simulink model "F18_Trim_2016b"  (R2016b)
settings: Solver=ode45  StartTime=0.0  StopTime=10.0  RelTol=1e-3  EnableMultiTasking=on
settings Model: Creator=mpc5200  LastModifiedBy=User
settings DataIOCC: LimitDataPoints=on  SaveFormat=Array  SignalLoggingSaveFormat=ModelDataLogs
settings OptimizationCC: ExpressionDepthLimit=2147483647  InitFltsAndDblsToZero=on  LifeSpan=inf
settings DebuggingCC: AlgebraicLoopMsg=none  SaveWithParameterizedLinksMsg=none  UnderspecifiedInitializationDetection=Classic  MergeDetectMultiDrivingBlocksExec=none  FcnCallInpInsideContextMsg=warning  UnconnectedInputMsg=none  UnconnectedOutputMsg=none  UnconnectedLineMsg=none  StateNameClashWarn=warning  SFUnexpectedBacktrackingDiag=warning  SFNoUnconditionalDefaultTransitionDiag=warning  SFExecutionAtInitializationDiag=none
settings HardwareCC: ProdBitPerPointer=32  ProdBitPerSizeT=32  ProdBitPerPtrDiffT=32  ProdLargestAtomicFloat=None  ProdIntDivRoundTo=Undefined  ProdEndianess=Unspecified  ProdWordSize=32  ProdHWDeviceType=32-bit Generic
settings ModelReferenceCC: PropagateSignalLabelsOutOfModel=off
settings GRTTargetCC: TargetFcnLib=ansi_tfl_tmw.mat  TargetLangStandard=C89/C90 (ANSI)  CombineOutputUpdateFcns=off  GRTInterface=on
settings ConfigComp: CovMetricSettings=dw  CovHtmlReporting=on  CovSaveCumulativeToWorkspaceVar=on  CovSaveSingleToWorkspaceVar=on  CovExternalEMLEnable=off

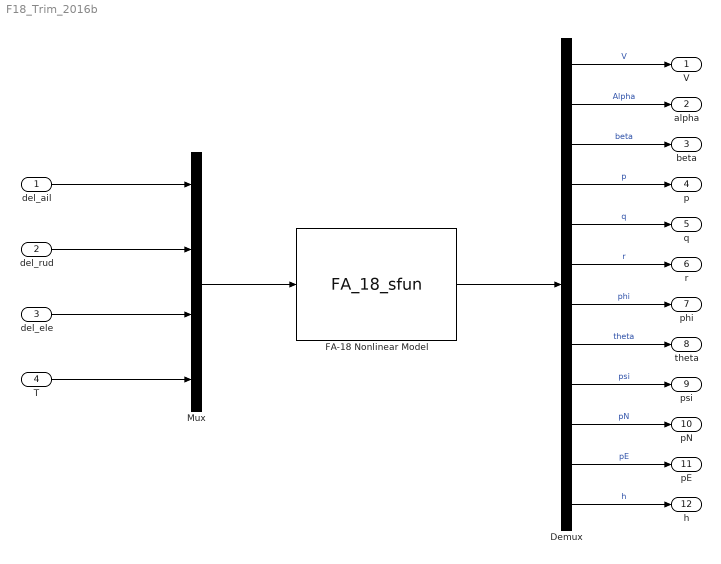
== system F18_Trim_2016b ==
  del_ail : Inport
  del_rud : Inport  Port=2
  del_ele : Inport  Port=3
  T : Inport  Port=4
  Demux : Demux  Outputs=12
  FA-18 Nonlinear Model : S-Function  FunctionName=FA_18_sfun  Parameters=x0  SFunctionDeploymentMode=off  EnableBusSupport=off
  Mux : Mux
  V : Outport
  alpha : Outport  Port=2
  beta : Outport  Port=3
  p : Outport  Port=4
  q : Outport  Port=5
  r : Outport  Port=6
  phi : Outport  Port=7
  theta : Outport  Port=8
  psi : Outport  Port=9
  pN : Outport  Port=10
  pE : Outport  Port=11
  h : Outport  Port=12
  wires:
  FA-18 Nonlinear Model/1 -> Demux/1
  Demux/2 -> alpha/1  "Alpha"
  Demux/7 -> phi/1  "phi"
  Demux/9 -> psi/1  "psi"
  Demux/12 -> h/1  "h"
  Demux/10 -> pN/1  "pN"
  Demux/3 -> beta/1  "beta"
  Demux/1 -> V/1  "V"
  Demux/8 -> theta/1  "theta"
  Demux/11 -> pE/1  "pE"
  Demux/5 -> q/1  "q"
  Demux/6 -> r/1  "r"
  Demux/4 -> p/1  "p"
  Mux/1 -> FA-18 Nonlinear Model/1
  del_ail/1 -> Mux/1
  del_rud/1 -> Mux/2
  del_ele/1 -> Mux/3
  T/1 -> Mux/4
